simulink model "ModelRiki"  (R2020a)
settings: Solver=ode45  StartTime=0.0  StopTime=inf  MaxStep=Ts  RelTol=1e-3  EnableMultiTasking=on
model workspace (MAT data in the model file):
  CG : Simulink.Parameter (value not decoded)
  GPSLL : Simulink.Parameter (value not decoded)
  Inertia : Simulink.Parameter (value not decoded)
  Mass : Simulink.Parameter (value not decoded)
  Ts : Simulink.Parameter (value not decoded)
values from neighbouring files (symbols this model uses):
  AltKp = 0.03    [params.mat]
  AltRateBias = 0.65    [params.mat]
  AltRateKi = 0.01    [params.mat]
  AltRateKp = 0.05    [params.mat]
  AltRateMax = 6    [params.mat]
  FilterK = [0.01 0.01 0.01 0.01 0.01 0.01 0.01 0.01 0.01 0.01 0.01 0.01 ... (100 elements, 1x100)]    [params.mat]
  PosKp = 0.1    [params.mat]
  RollPitchKp = 10    [params.mat]
  RollPitchMax = 30    [params.mat]
  RollPitchRateKd = 5e-05    [params.mat]
  RollPitchRateKi = 0.002    [params.mat]
  RollPitchRateKp = 0.0007    [params.mat]
  RollPitchRateMax = 200    [params.mat]
  VelKi = 0.02    [params.mat]
  VelKp = 0.15    [params.mat]
  VelMax = 6    [params.mat]
  Waypts = [10 20 50 50 50 50 200 20 20 0 0 50 ... (27 elements, 9x3)]    [params.mat]
  YawKp = 3    [params.mat]
  YawRateKi = 0.000213867089849    [params.mat]
  YawRateKp = 0.00321759853461    [params.mat]
  YawRateMax = 180    [params.mat]
symbols that are objects in the model workspace (value not decoded): CG, Mass, Ts
undefined symbols (not defined in the file or in its folder): AltRateKd, DiscIntNeverNeededParam, Earth, Receive, Send, sigbuilder_block, WGS84
libraries: simulink x50, sharedutil x8, simulink_extras x7, aerolibfltsims x5, aerolibanimutils x2, aerolibtransform2 x2, aerolibconvert2 x2, shared6dof x1, aerolibatmos2 x1
(part 4 of 4)

== system ModelRiki/Model/Landing Gears/W2 Wheel ==
  Model BUS : Inport
  TerrainHeight : Inport  Port=2
  Add : Sum
  Add1 : Sum  Inputs=|++
  Bus Selector : BusSelector  OutputSignals=DCM,Xe
  Compare To Constant : simulink/Logic and Bit Operations/Compare To Constant  relop=>=  const=0  OutDataTypeStr=uint8
  Display : Display
  Display1 : Display
  Display2 : Display
  Enabled Subsystem : Subsystem  TreatAsAtomicUnit=on
  Gear Location (Body) : Constant  Value=WheelLoc
  Matrix Multiply : Product  Multiplication=Matrix(*)
  Reshape : Reshape  OutputDimensionality=Row vector (2-D)
  Selector : Selector  InputPortWidth=3  IndexOptions=Index vector (dialog)  Indices=[3]  OutputSizes=1
  M[Nm] : Outport
  F[N] : Outport  Port=2
  wires:
  TerrainHeight/1 -> Add1/2
  Add1/1 -> Compare To Constant/1, Enabled Subsystem/1(Height)
  Selector/1 -> Add1/1
  Model BUS/1 -> Bus Selector/1
  Enabled Subsystem/2(M[Nm]) -> Display2/1, M[Nm]/1
  Enabled Subsystem/1(F[N]) -> Display1/1, F[N]/1
  Compare To Constant/1 -> Enabled Subsystem/Enable
  Reshape/1 -> Matrix Multiply/1
  Add/1 -> Selector/1, Display/1  "locationNED"
  Matrix Multiply/1 -> Add/1
  Gear Location (Body)/1 -> Reshape/1
  Bus Selector/2 -> Add/2  "<Xe>"
  Bus Selector/1 -> Matrix Multiply/2  "<DCM>"

== system ModelRiki/Model/Landing Gears/W3 Wheel ==
  Model BUS : Inport
  TerrainHeight : Inport  Port=2
  Add : Sum
  Add1 : Sum  Inputs=|++
  Bus Selector : BusSelector  OutputSignals=DCM,Xe
  Compare To Constant : simulink/Logic and Bit Operations/Compare To Constant  relop=>=  const=0  OutDataTypeStr=uint8
  Display : Display
  Display1 : Display
  Display2 : Display
  Enabled Subsystem : Subsystem  TreatAsAtomicUnit=on
  Gear Location (Body) : Constant  Value=WheelLoc
  Matrix Multiply : Product  Multiplication=Matrix(*)
  Reshape : Reshape  OutputDimensionality=Row vector (2-D)
  Selector : Selector  InputPortWidth=3  IndexOptions=Index vector (dialog)  Indices=[3]  OutputSizes=1
  M[Nm] : Outport
  F[N] : Outport  Port=2
  wires:
  Bus Selector/1 -> Matrix Multiply/2  "<DCM>"
  Bus Selector/2 -> Add/2  "<Xe>"
  Gear Location (Body)/1 -> Reshape/1
  Matrix Multiply/1 -> Add/1
  Add/1 -> Display/1, Selector/1  "locationNED"
  Reshape/1 -> Matrix Multiply/1
  Compare To Constant/1 -> Enabled Subsystem/Enable
  Enabled Subsystem/1(F[N]) -> F[N]/1, Display1/1
  Enabled Subsystem/2(M[Nm]) -> M[Nm]/1, Display2/1
  Model BUS/1 -> Bus Selector/1
  Selector/1 -> Add1/1
  Add1/1 -> Enabled Subsystem/1(Height), Compare To Constant/1
  TerrainHeight/1 -> Add1/2

== system ModelRiki/Model/Landing Gears/W4 Wheel ==
  Model BUS : Inport
  TerrainHeight : Inport  Port=2
  Add : Sum
  Add1 : Sum  Inputs=|++
  Bus Selector : BusSelector  OutputSignals=DCM,Xe
  Compare To Constant : simulink/Logic and Bit Operations/Compare To Constant  relop=>=  const=0  OutDataTypeStr=uint8
  Display : Display
  Display1 : Display
  Display2 : Display
  Enabled Subsystem : Subsystem  TreatAsAtomicUnit=on
  Gear Location (Body) : Constant  Value=WheelLoc
  Matrix Multiply : Product  Multiplication=Matrix(*)
  Reshape : Reshape  OutputDimensionality=Row vector (2-D)
  Selector : Selector  InputPortWidth=3  IndexOptions=Index vector (dialog)  Indices=[3]  OutputSizes=1
  M[Nm] : Outport
  F[N] : Outport  Port=2
  wires:
  TerrainHeight/1 -> Add1/2
  Add1/1 -> Compare To Constant/1, Enabled Subsystem/1(Height)
  Selector/1 -> Add1/1
  Model BUS/1 -> Bus Selector/1
  Enabled Subsystem/2(M[Nm]) -> Display2/1, M[Nm]/1
  Enabled Subsystem/1(F[N]) -> Display1/1, F[N]/1
  Compare To Constant/1 -> Enabled Subsystem/Enable
  Reshape/1 -> Matrix Multiply/1
  Add/1 -> Selector/1, Display/1  "locationNED"
  Matrix Multiply/1 -> Add/1
  Gear Location (Body)/1 -> Reshape/1
  Bus Selector/2 -> Add/2  "<Xe>"
  Bus Selector/1 -> Matrix Multiply/2  "<DCM>"

== system ModelRiki/Model/Propulsion/Motor1 ==
  InputPWM : Inport
  3x3 Cross Product : sharedutil/3x3 Cross Product  aMode=aMode
      settings: SourceProductBaseCode=AE,PW,MT,VE,VP
  Add : Sum  Inputs=+-
  Add1 : Sum  Inputs=|++
  Constant1 : Constant  Value="[0.159 -0.159  -0.05]"
  Constant2 : Constant  Value=CG
  Product : Product  RndMeth=Zero
  Product1 : Product  RndMeth=Zero
  Subsystem : Subsystem
  Terminator1 : Terminator
  Vector : Constant  Value=[0 0 -1]
  Vector1 : Constant  Value=[0 0 -1.0]
  F[N] : Outport
  M[Nm] : Outport  Port=2
  Current[A] : Outport  Port=3
  wires:
  Vector/1 -> Product/1  "Forcevector"
  Product/1 -> 3x3 Cross Product/2, F[N]/1
  Add/1 -> 3x3 Cross Product/1  "r"
  Constant1/1 -> Add/1  "Position"
  Constant2/1 -> Add/2  "CG"
  Subsystem/1(Thrust) -> Product/2
  InputPWM/1 -> Subsystem/1(PWM)
  3x3 Cross Product/1 -> Add1/1  "M"
  Add1/1 -> M[Nm]/1
  Product1/1 -> Add1/2  "RotorTorque"
  Subsystem/2(Torque) -> Product1/2
  Vector1/1 -> Product1/1
  Subsystem/3(Current) -> Current[A]/1
  Subsystem/4(RPM) -> Terminator1/1

== system ModelRiki/Model/Propulsion/Motor2 ==
  InputPWM : Inport
  3x3 Cross Product : sharedutil/3x3 Cross Product  aMode=aMode
      settings: SourceProductBaseCode=AE,PW,MT,VE,VP
  Add : Sum  Inputs=+-
  Add1 : Sum  Inputs=|++
  Constant1 : Constant  Value="[0.159 0.159  -0.05]"
  Constant2 : Constant  Value=CG
  Product : Product  RndMeth=Zero
  Product1 : Product  RndMeth=Zero
  Subsystem : Subsystem
  Terminator1 : Terminator
  Vector : Constant  Value=[0 0 -1]
  Vector1 : Constant  Value=[0 0 1.0]
  F[N] : Outport
  M[Nm] : Outport  Port=2
  Current[A] : Outport  Port=3
  wires:
  Vector/1 -> Product/1  "Forcevector"
  Product/1 -> 3x3 Cross Product/2, F[N]/1
  Add/1 -> 3x3 Cross Product/1  "r"
  Constant1/1 -> Add/1  "Position"
  Constant2/1 -> Add/2  "CG"
  Subsystem/1(Thrust) -> Product/2
  InputPWM/1 -> Subsystem/1(PWM)
  3x3 Cross Product/1 -> Add1/1  "M"
  Add1/1 -> M[Nm]/1
  Product1/1 -> Add1/2  "RotorTorque"
  Subsystem/2(Torque) -> Product1/2
  Vector1/1 -> Product1/1
  Subsystem/3(Current) -> Current[A]/1
  Subsystem/4(RPM) -> Terminator1/1

== system ModelRiki/Model/Propulsion/Motor3 ==
  InputPWM : Inport
  3x3 Cross Product : sharedutil/3x3 Cross Product  aMode=aMode
      settings: SourceProductBaseCode=AE,PW,MT,VE,VP
  Add : Sum  Inputs=+-
  Add1 : Sum  Inputs=|++
  Constant1 : Constant  Value="[-0.159 0.159  -0.05]"
  Constant2 : Constant  Value=CG
  Product : Product  RndMeth=Zero
  Product1 : Product  RndMeth=Zero
  Subsystem : Subsystem
  Terminator1 : Terminator
  Vector : Constant  Value=[0 0 -1]
  Vector1 : Constant  Value=[0 0 -1.0]
  F[N] : Outport
  M[Nm] : Outport  Port=2
  Current[A] : Outport  Port=3
  wires:
  Vector/1 -> Product/1  "Forcevector"
  Product/1 -> 3x3 Cross Product/2, F[N]/1
  Add/1 -> 3x3 Cross Product/1  "r"
  Constant1/1 -> Add/1  "Position"
  Constant2/1 -> Add/2  "CG"
  Subsystem/1(Thrust) -> Product/2
  InputPWM/1 -> Subsystem/1(PWM)
  3x3 Cross Product/1 -> Add1/1  "M"
  Add1/1 -> M[Nm]/1
  Product1/1 -> Add1/2  "RotorTorque"
  Subsystem/2(Torque) -> Product1/2
  Vector1/1 -> Product1/1
  Subsystem/3(Current) -> Current[A]/1
  Subsystem/4(RPM) -> Terminator1/1

== system ModelRiki/Model/Propulsion/Motor4 ==
  InputPWM : Inport
  3x3 Cross Product : sharedutil/3x3 Cross Product  aMode=aMode
      settings: SourceProductBaseCode=AE,PW,MT,VE,VP
  Add : Sum  Inputs=+-
  Add1 : Sum  Inputs=|++
  Constant1 : Constant  Value="[-0.159 -0.159  -0.05]"
  Constant2 : Constant  Value=CG
  Product : Product  RndMeth=Zero
  Product1 : Product  RndMeth=Zero
  Subsystem : Subsystem
  Terminator1 : Terminator
  Vector : Constant  Value=[0 0 -1]
  Vector1 : Constant  Value=[0 0 1.0]
  F[N] : Outport
  M[Nm] : Outport  Port=2
  Current[A] : Outport  Port=3
  wires:
  Vector/1 -> Product/1  "Forcevector"
  Product/1 -> 3x3 Cross Product/2, F[N]/1
  Add/1 -> 3x3 Cross Product/1  "r"
  Constant1/1 -> Add/1  "Position"
  Constant2/1 -> Add/2  "CG"
  Subsystem/1(Thrust) -> Product/2
  InputPWM/1 -> Subsystem/1(PWM)
  3x3 Cross Product/1 -> Add1/1  "M"
  Add1/1 -> M[Nm]/1
  Product1/1 -> Add1/2  "RotorTorque"
  Subsystem/2(Torque) -> Product1/2
  Vector1/1 -> Product1/1
  Subsystem/3(Current) -> Current[A]/1
  Subsystem/4(RPM) -> Terminator1/1

== system ModelRiki/Ctrl/AutoCtrl/Mapper/LimitAndRescale ==
  Scaled : Inport
  Constant : Constant  Value=1100  OutDataTypeStr=single
  Gain : Gain  Gain=(1900-1100)
  Limit3 : Saturate  UpperLimit=1  LowerLimit=0
  Subtract : Sum
  ESCPWM : Outport
  wires:
  Constant/1 -> Subtract/2
  Gain/1 -> Subtract/1
  Scaled/1 -> Limit3/1
  Subtract/1 -> ESCPWM/1
  Limit3/1 -> Gain/1

== system ModelRiki/Ctrl/AutoCtrl/Mapper/LimitAndRescale1 ==
  Scaled : Inport
  Constant : Constant  Value=1100  OutDataTypeStr=single
  Gain : Gain  Gain=(1900-1100)
  Limit3 : Saturate  UpperLimit=1  LowerLimit=0
  Subtract : Sum
  ESCPWM : Outport
  wires:
  Constant/1 -> Subtract/2
  Gain/1 -> Subtract/1
  Scaled/1 -> Limit3/1
  Subtract/1 -> ESCPWM/1
  Limit3/1 -> Gain/1

== system ModelRiki/Ctrl/AutoCtrl/Mapper/LimitAndRescale2 ==
  Scaled : Inport
  Constant : Constant  Value=1100  OutDataTypeStr=single
  Gain : Gain  Gain=(1900-1100)
  Limit3 : Saturate  UpperLimit=1  LowerLimit=0
  Subtract : Sum
  ESCPWM : Outport
  wires:
  Constant/1 -> Subtract/2
  Gain/1 -> Subtract/1
  Scaled/1 -> Limit3/1
  Subtract/1 -> ESCPWM/1
  Limit3/1 -> Gain/1

== system ModelRiki/Ctrl/AutoCtrl/Mapper/LimitAndRescale3 ==
  Scaled : Inport
  Constant : Constant  Value=1100  OutDataTypeStr=single
  Gain : Gain  Gain=(1900-1100)
  Limit3 : Saturate  UpperLimit=1  LowerLimit=0
  Subtract : Sum
  ESCPWM : Outport
  wires:
  Constant/1 -> Subtract/2
  Gain/1 -> Subtract/1
  Scaled/1 -> Limit3/1
  Subtract/1 -> ESCPWM/1
  Limit3/1 -> Gain/1

== system ModelRiki/Ctrl/ManualCtrl/Mapper/LimitAndRescale ==
  Scaled : Inport
  Constant : Constant  Value=1100  OutDataTypeStr=single
  Gain : Gain  Gain=(1900-1100)
  Limit3 : Saturate  UpperLimit=1  LowerLimit=0
  Subtract : Sum
  ESCPWM : Outport
  wires:
  Constant/1 -> Subtract/2
  Gain/1 -> Subtract/1
  Scaled/1 -> Limit3/1
  Subtract/1 -> ESCPWM/1
  Limit3/1 -> Gain/1

== system ModelRiki/Ctrl/ManualCtrl/Mapper/LimitAndRescale1 ==
  Scaled : Inport
  Constant : Constant  Value=1100  OutDataTypeStr=single
  Gain : Gain  Gain=(1900-1100)
  Limit3 : Saturate  UpperLimit=1  LowerLimit=0
  Subtract : Sum
  ESCPWM : Outport
  wires:
  Constant/1 -> Subtract/2
  Gain/1 -> Subtract/1
  Scaled/1 -> Limit3/1
  Subtract/1 -> ESCPWM/1
  Limit3/1 -> Gain/1

== system ModelRiki/Ctrl/ManualCtrl/Mapper/LimitAndRescale2 ==
  Scaled : Inport
  Constant : Constant  Value=1100  OutDataTypeStr=single
  Gain : Gain  Gain=(1900-1100)
  Limit3 : Saturate  UpperLimit=1  LowerLimit=0
  Subtract : Sum
  ESCPWM : Outport
  wires:
  Constant/1 -> Subtract/2
  Gain/1 -> Subtract/1
  Scaled/1 -> Limit3/1
  Subtract/1 -> ESCPWM/1
  Limit3/1 -> Gain/1

== system ModelRiki/Ctrl/ManualCtrl/Mapper/LimitAndRescale3 ==
  Scaled : Inport
  Constant : Constant  Value=1100  OutDataTypeStr=single
  Gain : Gain  Gain=(1900-1100)
  Limit3 : Saturate  UpperLimit=1  LowerLimit=0
  Subtract : Sum
  ESCPWM : Outport
  wires:
  Constant/1 -> Subtract/2
  Gain/1 -> Subtract/1
  Scaled/1 -> Limit3/1
  Subtract/1 -> ESCPWM/1
  Limit3/1 -> Gain/1

== system ModelRiki/Ctrl/RateCtrl/Mapper/LimitAndRescale ==
  Scaled : Inport
  Constant : Constant  Value=1100  OutDataTypeStr=single
  Gain : Gain  Gain=(1900-1100)
  Limit3 : Saturate  UpperLimit=1  LowerLimit=0
  Subtract : Sum
  ESCPWM : Outport
  wires:
  Constant/1 -> Subtract/2
  Gain/1 -> Subtract/1
  Scaled/1 -> Limit3/1
  Subtract/1 -> ESCPWM/1
  Limit3/1 -> Gain/1

== system ModelRiki/Ctrl/RateCtrl/Mapper/LimitAndRescale1 ==
  Scaled : Inport
  Constant : Constant  Value=1100  OutDataTypeStr=single
  Gain : Gain  Gain=(1900-1100)
  Limit3 : Saturate  UpperLimit=1  LowerLimit=0
  Subtract : Sum
  ESCPWM : Outport
  wires:
  Constant/1 -> Subtract/2
  Gain/1 -> Subtract/1
  Scaled/1 -> Limit3/1
  Subtract/1 -> ESCPWM/1
  Limit3/1 -> Gain/1

== system ModelRiki/Ctrl/RateCtrl/Mapper/LimitAndRescale2 ==
  Scaled : Inport
  Constant : Constant  Value=1100  OutDataTypeStr=single
  Gain : Gain  Gain=(1900-1100)
  Limit3 : Saturate  UpperLimit=1  LowerLimit=0
  Subtract : Sum
  ESCPWM : Outport
  wires:
  Constant/1 -> Subtract/2
  Gain/1 -> Subtract/1
  Scaled/1 -> Limit3/1
  Subtract/1 -> ESCPWM/1
  Limit3/1 -> Gain/1

== system ModelRiki/Ctrl/RateCtrl/Mapper/LimitAndRescale3 ==
  Scaled : Inport
  Constant : Constant  Value=1100  OutDataTypeStr=single
  Gain : Gain  Gain=(1900-1100)
  Limit3 : Saturate  UpperLimit=1  LowerLimit=0
  Subtract : Sum
  ESCPWM : Outport
  wires:
  Constant/1 -> Subtract/2
  Gain/1 -> Subtract/1
  Scaled/1 -> Limit3/1
  Subtract/1 -> ESCPWM/1
  Limit3/1 -> Gain/1

== system ModelRiki/Ctrl/RollPitchCtrl/Mapper/LimitAndRescale ==
  Scaled : Inport
  Constant : Constant  Value=1100  OutDataTypeStr=single
  Gain : Gain  Gain=(1900-1100)
  Limit3 : Saturate  UpperLimit=1  LowerLimit=0
  Subtract : Sum
  ESCPWM : Outport
  wires:
  Constant/1 -> Subtract/2
  Gain/1 -> Subtract/1
  Scaled/1 -> Limit3/1
  Subtract/1 -> ESCPWM/1
  Limit3/1 -> Gain/1

== system ModelRiki/Ctrl/RollPitchCtrl/Mapper/LimitAndRescale1 ==
  Scaled : Inport
  Constant : Constant  Value=1100  OutDataTypeStr=single
  Gain : Gain  Gain=(1900-1100)
  Limit3 : Saturate  UpperLimit=1  LowerLimit=0
  Subtract : Sum
  ESCPWM : Outport
  wires:
  Constant/1 -> Subtract/2
  Gain/1 -> Subtract/1
  Scaled/1 -> Limit3/1
  Subtract/1 -> ESCPWM/1
  Limit3/1 -> Gain/1

== system ModelRiki/Ctrl/RollPitchCtrl/Mapper/LimitAndRescale2 ==
  Scaled : Inport
  Constant : Constant  Value=1100  OutDataTypeStr=single
  Gain : Gain  Gain=(1900-1100)
  Limit3 : Saturate  UpperLimit=1  LowerLimit=0
  Subtract : Sum
  ESCPWM : Outport
  wires:
  Constant/1 -> Subtract/2
  Gain/1 -> Subtract/1
  Scaled/1 -> Limit3/1
  Subtract/1 -> ESCPWM/1
  Limit3/1 -> Gain/1

== system ModelRiki/Ctrl/RollPitchCtrl/Mapper/LimitAndRescale3 ==
  Scaled : Inport
  Constant : Constant  Value=1100  OutDataTypeStr=single
  Gain : Gain  Gain=(1900-1100)
  Limit3 : Saturate  UpperLimit=1  LowerLimit=0
  Subtract : Sum
  ESCPWM : Outport
  wires:
  Constant/1 -> Subtract/2
  Gain/1 -> Subtract/1
  Scaled/1 -> Limit3/1
  Subtract/1 -> ESCPWM/1
  Limit3/1 -> Gain/1

== system ModelRiki/Ctrl/VelocityCtrl/Mapper/LimitAndRescale ==
  Scaled : Inport
  Constant : Constant  Value=1100  OutDataTypeStr=single
  Gain : Gain  Gain=(1900-1100)
  Limit3 : Saturate  UpperLimit=1  LowerLimit=0
  Subtract : Sum
  ESCPWM : Outport
  wires:
  Constant/1 -> Subtract/2
  Gain/1 -> Subtract/1
  Scaled/1 -> Limit3/1
  Subtract/1 -> ESCPWM/1
  Limit3/1 -> Gain/1

== system ModelRiki/Ctrl/VelocityCtrl/Mapper/LimitAndRescale1 ==
  Scaled : Inport
  Constant : Constant  Value=1100  OutDataTypeStr=single
  Gain : Gain  Gain=(1900-1100)
  Limit3 : Saturate  UpperLimit=1  LowerLimit=0
  Subtract : Sum
  ESCPWM : Outport
  wires:
  Constant/1 -> Subtract/2
  Gain/1 -> Subtract/1
  Scaled/1 -> Limit3/1
  Subtract/1 -> ESCPWM/1
  Limit3/1 -> Gain/1

== system ModelRiki/Ctrl/VelocityCtrl/Mapper/LimitAndRescale2 ==
  Scaled : Inport
  Constant : Constant  Value=1100  OutDataTypeStr=single
  Gain : Gain  Gain=(1900-1100)
  Limit3 : Saturate  UpperLimit=1  LowerLimit=0
  Subtract : Sum
  ESCPWM : Outport
  wires:
  Constant/1 -> Subtract/2
  Gain/1 -> Subtract/1
  Scaled/1 -> Limit3/1
  Subtract/1 -> ESCPWM/1
  Limit3/1 -> Gain/1

== system ModelRiki/Ctrl/VelocityCtrl/Mapper/LimitAndRescale3 ==
  Scaled : Inport
  Constant : Constant  Value=1100  OutDataTypeStr=single
  Gain : Gain  Gain=(1900-1100)
  Limit3 : Saturate  UpperLimit=1  LowerLimit=0
  Subtract : Sum
  ESCPWM : Outport
  wires:
  Constant/1 -> Subtract/2
  Gain/1 -> Subtract/1
  Scaled/1 -> Limit3/1
  Subtract/1 -> ESCPWM/1
  Limit3/1 -> Gain/1

== system ModelRiki/Model/Landing Gears/W1 Wheel/Enabled Subsystem ==
  Height : Inport
  Enable : EnablePort
  3x3 Cross Product : sharedutil/3x3 Cross Product  aMode=aMode
      settings: SourceProductBaseCode=AE,PW,MT,VE,VP
  Add : Sum  Inputs=+-
  Add1 : Sum
  Constant2 : Constant  Value=CG
  Derivative : Derivative
  Gain : Gain  Gain=1000
  Gain1 : Gain  Gain=200
  Gear Location (Body) : Constant  Value=WheelLoc
  Gear Vector (up) : Constant  Value=[0 0 -1]
  Product : Product  RndMeth=Zero
  F[N] : Outport  OutputWhenDisabled=reset  InitialOutput=[0 0 0]
  M[Nm] : Outport  Port=2  OutputWhenDisabled=reset  InitialOutput=[0 0 0]
  wires:
  Product/1 -> 3x3 Cross Product/2, F[N]/1
  Add/1 -> 3x3 Cross Product/1  "r"
  Gear Location (Body)/1 -> Add/1  "Position"
  Constant2/1 -> Add/2  "CG"
  Gear Vector (up)/1 -> Product/1
  3x3 Cross Product/1 -> M[Nm]/1  "M"
  Height/1 -> Gain/1, Derivative/1
  Add1/1 -> Product/2
  Gain/1 -> Add1/1
  Derivative/1 -> Gain1/1
  Gain1/1 -> Add1/2

== system ModelRiki/Model/Landing Gears/W2 Wheel/Enabled Subsystem ==
  Height : Inport
  Enable : EnablePort
  3x3 Cross Product : sharedutil/3x3 Cross Product  aMode=aMode
      settings: SourceProductBaseCode=AE,PW,MT,VE,VP
  Add : Sum  Inputs=+-
  Add1 : Sum
  Constant2 : Constant  Value=CG
  Derivative : Derivative
  Gain : Gain  Gain=1000
  Gain1 : Gain  Gain=200
  Gear Location (Body) : Constant  Value=WheelLoc
  Gear Vector (up) : Constant  Value=[0 0 -1]
  Product : Product  RndMeth=Zero
  F[N] : Outport  OutputWhenDisabled=reset  InitialOutput=[0 0 0]
  M[Nm] : Outport  Port=2  OutputWhenDisabled=reset  InitialOutput=[0 0 0]
  wires:
  Gain1/1 -> Add1/2
  Derivative/1 -> Gain1/1
  Gain/1 -> Add1/1
  Add1/1 -> Product/2
  Height/1 -> Derivative/1, Gain/1
  3x3 Cross Product/1 -> M[Nm]/1  "M"
  Gear Vector (up)/1 -> Product/1
  Constant2/1 -> Add/2  "CG"
  Gear Location (Body)/1 -> Add/1  "Position"
  Add/1 -> 3x3 Cross Product/1  "r"
  Product/1 -> F[N]/1, 3x3 Cross Product/2

== system ModelRiki/Model/Landing Gears/W3 Wheel/Enabled Subsystem ==
  Height : Inport
  Enable : EnablePort
  3x3 Cross Product : sharedutil/3x3 Cross Product  aMode=aMode
      settings: SourceProductBaseCode=AE,PW,MT,VE,VP
  Add : Sum  Inputs=+-
  Add1 : Sum
  Constant2 : Constant  Value=CG
  Derivative : Derivative
  Gain : Gain  Gain=1000
  Gain1 : Gain  Gain=200
  Gear Location (Body) : Constant  Value=WheelLoc
  Gear Vector (up) : Constant  Value=[0 0 -1]
  Product : Product  RndMeth=Zero
  F[N] : Outport  OutputWhenDisabled=reset  InitialOutput=[0 0 0]
  M[Nm] : Outport  Port=2  OutputWhenDisabled=reset  InitialOutput=[0 0 0]
  wires:
  Product/1 -> 3x3 Cross Product/2, F[N]/1
  Add/1 -> 3x3 Cross Product/1  "r"
  Gear Location (Body)/1 -> Add/1  "Position"
  Constant2/1 -> Add/2  "CG"
  Gear Vector (up)/1 -> Product/1
  3x3 Cross Product/1 -> M[Nm]/1  "M"
  Height/1 -> Gain/1, Derivative/1
  Add1/1 -> Product/2
  Gain/1 -> Add1/1
  Derivative/1 -> Gain1/1
  Gain1/1 -> Add1/2

== system ModelRiki/Model/Landing Gears/W4 Wheel/Enabled Subsystem ==
  Height : Inport
  Enable : EnablePort
  3x3 Cross Product : sharedutil/3x3 Cross Product  aMode=aMode
      settings: SourceProductBaseCode=AE,PW,MT,VE,VP
  Add : Sum  Inputs=+-
  Add1 : Sum
  Constant2 : Constant  Value=CG
  Derivative : Derivative
  Gain : Gain  Gain=1000
  Gain1 : Gain  Gain=200
  Gear Location (Body) : Constant  Value=WheelLoc
  Gear Vector (up) : Constant  Value=[0 0 -1]
  Product : Product  RndMeth=Zero
  F[N] : Outport  OutputWhenDisabled=reset  InitialOutput=[0 0 0]
  M[Nm] : Outport  Port=2  OutputWhenDisabled=reset  InitialOutput=[0 0 0]
  wires:
  Gain1/1 -> Add1/2
  Derivative/1 -> Gain1/1
  Gain/1 -> Add1/1
  Add1/1 -> Product/2
  Height/1 -> Derivative/1, Gain/1
  3x3 Cross Product/1 -> M[Nm]/1  "M"
  Gear Vector (up)/1 -> Product/1
  Constant2/1 -> Add/2  "CG"
  Gear Location (Body)/1 -> Add/1  "Position"
  Add/1 -> 3x3 Cross Product/1  "r"
  Product/1 -> F[N]/1, 3x3 Cross Product/2

== system ModelRiki/Model/Propulsion/Motor1/Subsystem ==
  note: [N]
  note: [g]
  note: [Nm]
  note: [A]
  note: [20ms delay?]
  note: [Torque estimated]
  note: [1000-1900]
  note: Current
  note: Enable [>1150]
  PWM : Inport  OutDataTypeStr=double  PortDimensions=1  SampleTime=0
  Compare To Constant1 : simulink/Logic and Bit Operations/Compare To Constant  relop=>=  const=1150  OutDataTypeStr=boolean
  Constant1 : Constant  Value=0
  Gain2 : Gain  Gain=1/1000
  Gain3 : Gain  Gain=1/1000*9.81
  Polynomial4 : Polyval  Coefs="[194.0242  232.6928 -846.8342  374.2523]"
  Polynomial5 : Polyval  Coefs="[23.1858  -80.9421   97.9875  -40.9978]"
  Polynomial6 : Polyval  Coefs="1.0e+04 *[-0.6016    2.6561   -2.8627    0.8887]"
  Polynomial7 : Polyval  Coefs="1e-3*0.11*[194.0242  232.6928 -846.8342  374.2523]"
  Saturation1 : Saturate  UpperLimit=1900  LowerLimit=1000
  Switch{4..7} (4 alike) : Switch  Criteria=u2 ~= 0
  Transfer Fcn1 : TransferFcn  Denominator=[0.045 1]
  Transport Delay1 : TransportDelay  DelayTime=0.02
  Thrust : Outport  OutDataTypeStr=double  PortDimensions=1  SampleTime=0
  Torque : Outport  Port=2  OutDataTypeStr=double  PortDimensions=1  SampleTime=0
  Current : Outport  Port=3  OutDataTypeStr=double  PortDimensions=1  SampleTime=0
  RPM : Outport  Port=4  OutDataTypeStr=double  PortDimensions=1  SampleTime=0
  wires:
  Gain3/1 -> Thrust/1  "Thrust"
  Saturation1/1 -> Transport Delay1/1
  Transport Delay1/1 -> Transfer Fcn1/1
  Gain2/1 -> Polynomial4/1, Polynomial6/1, Polynomial5/1, Polynomial7/1
  Compare To Constant1/1 -> Switch4/2, Switch6/2, Switch5/2, Switch7/2
  Polynomial4/1 -> Switch4/1
  Constant1/1 -> Switch4/3, Switch6/3, Switch5/3, Switch7/3
  Switch4/1 -> Gain3/1  "Thrust"
  Polynomial5/1 -> Switch5/1
  Switch5/1 -> Current/1
  Polynomial6/1 -> Switch6/1
  Switch6/1 -> RPM/1  "RPM"
  Polynomial7/1 -> Switch7/1
  Switch7/1 -> Torque/1  "Torque"
  Transfer Fcn1/1 -> Gain2/1, Compare To Constant1/1
  PWM/1 -> Saturation1/1

== system ModelRiki/Model/Propulsion/Motor2/Subsystem ==
  note: [N]
  note: [g]
  note: [Nm]
  note: [A]
  note: [20ms delay?]
  note: [Torque estimated]
  note: [1000-1900]
  note: Current
  note: Enable [>1150]
  PWM : Inport  OutDataTypeStr=double  PortDimensions=1  SampleTime=0
  Compare To Constant1 : simulink/Logic and Bit Operations/Compare To Constant  relop=>=  const=1150  OutDataTypeStr=boolean
  Constant1 : Constant  Value=0
  Gain2 : Gain  Gain=1/1000
  Gain3 : Gain  Gain=1/1000*9.81
  Polynomial4 : Polyval  Coefs="[194.0242  232.6928 -846.8342  374.2523]"
  Polynomial5 : Polyval  Coefs="[23.1858  -80.9421   97.9875  -40.9978]"
  Polynomial6 : Polyval  Coefs="1.0e+04 *[-0.6016    2.6561   -2.8627    0.8887]"
  Polynomial7 : Polyval  Coefs="1e-3*0.11*[194.0242  232.6928 -846.8342  374.2523]"
  Saturation1 : Saturate  UpperLimit=1900  LowerLimit=1000
  Switch{4..7} (4 alike) : Switch  Criteria=u2 ~= 0
  Transfer Fcn1 : TransferFcn  Denominator=[0.045 1]
  Transport Delay1 : TransportDelay  DelayTime=0.02
  Thrust : Outport  OutDataTypeStr=double  PortDimensions=1  SampleTime=0
  Torque : Outport  Port=2  OutDataTypeStr=double  PortDimensions=1  SampleTime=0
  Current : Outport  Port=3  OutDataTypeStr=double  PortDimensions=1  SampleTime=0
  RPM : Outport  Port=4  OutDataTypeStr=double  PortDimensions=1  SampleTime=0
  wires:
  Gain3/1 -> Thrust/1  "Thrust"
  Saturation1/1 -> Transport Delay1/1
  Transport Delay1/1 -> Transfer Fcn1/1
  Gain2/1 -> Polynomial4/1, Polynomial6/1, Polynomial5/1, Polynomial7/1
  Compare To Constant1/1 -> Switch4/2, Switch6/2, Switch5/2, Switch7/2
  Polynomial4/1 -> Switch4/1
  Constant1/1 -> Switch4/3, Switch6/3, Switch5/3, Switch7/3
  Switch4/1 -> Gain3/1  "Thrust"
  Polynomial5/1 -> Switch5/1
  Switch5/1 -> Current/1
  Polynomial6/1 -> Switch6/1
  Switch6/1 -> RPM/1  "RPM"
  Polynomial7/1 -> Switch7/1
  Switch7/1 -> Torque/1  "Torque"
  Transfer Fcn1/1 -> Gain2/1, Compare To Constant1/1
  PWM/1 -> Saturation1/1

== system ModelRiki/Model/Propulsion/Motor3/Subsystem ==
  note: [N]
  note: [g]
  note: [Nm]
  note: [A]
  note: [20ms delay?]
  note: [Torque estimated]
  note: [1000-1900]
  note: Current
  note: Enable [>1150]
  PWM : Inport  OutDataTypeStr=double  PortDimensions=1  SampleTime=0
  Compare To Constant1 : simulink/Logic and Bit Operations/Compare To Constant  relop=>=  const=1150  OutDataTypeStr=boolean
  Constant1 : Constant  Value=0
  Gain2 : Gain  Gain=1/1000
  Gain3 : Gain  Gain=1/1000*9.81
  Polynomial4 : Polyval  Coefs="[194.0242  232.6928 -846.8342  374.2523]"
  Polynomial5 : Polyval  Coefs="[23.1858  -80.9421   97.9875  -40.9978]"
  Polynomial6 : Polyval  Coefs="1.0e+04 *[-0.6016    2.6561   -2.8627    0.8887]"
  Polynomial7 : Polyval  Coefs="1e-3*0.11*[194.0242  232.6928 -846.8342  374.2523]"
  Saturation1 : Saturate  UpperLimit=1900  LowerLimit=1000
  Switch{4..7} (4 alike) : Switch  Criteria=u2 ~= 0
  Transfer Fcn1 : TransferFcn  Denominator=[0.045 1]
  Transport Delay1 : TransportDelay  DelayTime=0.02
  Thrust : Outport  OutDataTypeStr=double  PortDimensions=1  SampleTime=0
  Torque : Outport  Port=2  OutDataTypeStr=double  PortDimensions=1  SampleTime=0
  Current : Outport  Port=3  OutDataTypeStr=double  PortDimensions=1  SampleTime=0
  RPM : Outport  Port=4  OutDataTypeStr=double  PortDimensions=1  SampleTime=0
  wires:
  Gain3/1 -> Thrust/1  "Thrust"
  Saturation1/1 -> Transport Delay1/1
  Transport Delay1/1 -> Transfer Fcn1/1
  Gain2/1 -> Polynomial4/1, Polynomial6/1, Polynomial5/1, Polynomial7/1
  Compare To Constant1/1 -> Switch4/2, Switch6/2, Switch5/2, Switch7/2
  Polynomial4/1 -> Switch4/1
  Constant1/1 -> Switch4/3, Switch6/3, Switch5/3, Switch7/3
  Switch4/1 -> Gain3/1  "Thrust"
  Polynomial5/1 -> Switch5/1
  Switch5/1 -> Current/1
  Polynomial6/1 -> Switch6/1
  Switch6/1 -> RPM/1  "RPM"
  Polynomial7/1 -> Switch7/1
  Switch7/1 -> Torque/1  "Torque"
  Transfer Fcn1/1 -> Gain2/1, Compare To Constant1/1
  PWM/1 -> Saturation1/1

== system ModelRiki/Model/Propulsion/Motor4/Subsystem ==
  note: [N]
  note: [g]
  note: [Nm]
  note: [A]
  note: [20ms delay?]
  note: [Torque estimated]
  note: [1000-1900]
  note: Current
  note: Enable [>1150]
  PWM : Inport  OutDataTypeStr=double  PortDimensions=1  SampleTime=0
  Compare To Constant1 : simulink/Logic and Bit Operations/Compare To Constant  relop=>=  const=1150  OutDataTypeStr=boolean
  Constant1 : Constant  Value=0
  Gain2 : Gain  Gain=1/1000
  Gain3 : Gain  Gain=1/1000*9.81
  Polynomial4 : Polyval  Coefs="[194.0242  232.6928 -846.8342  374.2523]"
  Polynomial5 : Polyval  Coefs="[23.1858  -80.9421   97.9875  -40.9978]"
  Polynomial6 : Polyval  Coefs="1.0e+04 *[-0.6016    2.6561   -2.8627    0.8887]"
  Polynomial7 : Polyval  Coefs="1e-3*0.11*[194.0242  232.6928 -846.8342  374.2523]"
  Saturation1 : Saturate  UpperLimit=1900  LowerLimit=1000
  Switch{4..7} (4 alike) : Switch  Criteria=u2 ~= 0
  Transfer Fcn1 : TransferFcn  Denominator=[0.045 1]
  Transport Delay1 : TransportDelay  DelayTime=0.02
  Thrust : Outport  OutDataTypeStr=double  PortDimensions=1  SampleTime=0
  Torque : Outport  Port=2  OutDataTypeStr=double  PortDimensions=1  SampleTime=0
  Current : Outport  Port=3  OutDataTypeStr=double  PortDimensions=1  SampleTime=0
  RPM : Outport  Port=4  OutDataTypeStr=double  PortDimensions=1  SampleTime=0
  wires:
  Gain3/1 -> Thrust/1  "Thrust"
  Saturation1/1 -> Transport Delay1/1
  Transport Delay1/1 -> Transfer Fcn1/1
  Gain2/1 -> Polynomial4/1, Polynomial6/1, Polynomial5/1, Polynomial7/1
  Compare To Constant1/1 -> Switch4/2, Switch6/2, Switch5/2, Switch7/2
  Polynomial4/1 -> Switch4/1
  Constant1/1 -> Switch4/3, Switch6/3, Switch5/3, Switch7/3
  Switch4/1 -> Gain3/1  "Thrust"
  Polynomial5/1 -> Switch5/1
  Switch5/1 -> Current/1
  Polynomial6/1 -> Switch6/1
  Switch6/1 -> RPM/1  "RPM"
  Polynomial7/1 -> Switch7/1
  Switch7/1 -> Torque/1  "Torque"
  Transfer Fcn1/1 -> Gain2/1, Compare To Constant1/1
  PWM/1 -> Saturation1/1

== stateflow chart ModelRiki/Ctrl/Chart ==
  settings: updateMethod=DISCRETE  sampleTime=Ts
  state SystemLogic [parallel]
    en: Mode = uint8(0);
    du: SelectMode()
    settings: executionOrder=1
    state On
      en:
      ModeOld = Mode;
      state ManualMode
        entry:
        ActualMode=uint8(1);
      state RateMode
        entry:
        ActualMode=uint8(2);
      state RollPitchMode
        entry:
        ActualMode=uint8(3);
      state VelocityMode
        entry:
        ActualMode=uint8(4);
      state AutoMode
        state InitSegment
          entry:
          ActualMode=10+wayIndex;
          CalculateTrajSegment(wayIndex,wayIndex+1, TrajZNEVParams(4))
          Time = single(0);
          AutoRefAng = atan2(Waypoints(wayIndex+1,3)-Waypoints(wayIndex,3), Waypoints(wayIndex+1,2)-Waypoints(wayIndex,2) );
        state Idle
          entry:
          wayIndex = uint8(1);
          ActualMode=uint8(5);
          during:
          AutoRef=Waypoints(1,:); % Altitude, N, E
          AutoRefAng = single(-2000); % disable
        state GotoWaypoint
          during:
          AutoRef = P1 + dPdT*Time;
          Time = Time+Ts;
        state NextWaypoint
          entry:
          wayIndex=wayIndex+1;
        state End
        state Orbit
          during:
          AutoRef(1) = TrajZNEVParams(1);
          AutoRef(2) = TrajZNEVParams(2) + cos(OrbPhi) * OrbRadius;
          AutoRef(3) = TrajZNEVParams(3) + sin(OrbPhi) * OrbRadius;
          OrbPhi = OrbPhi+(OrbdPhidT*Ts);
          AutoRefAng = OrbPhi+pi;
          while AutoRefAng > 2*pi
          AutoRefAng = AutoRefAng-(2*pi);
          end
        state InitOrbitBezSecera
          entry:
          OrbRadius = sqrt( (Position(2) - TrajZNEVParams(2))^2 + (Position(3) - TrajZNEVParams(3))^2 );
          OrbPhi = atan2((Position(3) - TrajZNEVParams(3)), (Position(2) - TrajZNEVParams(2)));
          OrbdPhidT = TrajZNEVParams(4) / OrbRadius; % phi per second to match speed V
        GotoWaypoint -> Idle [order 2] : [ExecuteWaypoints == 10] % Abort Command
        (default) -> Idle
        InitSegment -> GotoWaypoint
        Idle -> InitSegment [order 1] : [ ExecuteWaypoints == 1 && (WayCnt > 0) ]
        Idle -> InitOrbitBezSecera [order 2] : [ ExecuteWaypoints == 2]
        GotoWaypoint -> NextWaypoint [order 1] : [Time > Ttotal]
        End -> Idle
        (junction 284) -> InitSegment [order 2]
        (junction 284) -> End [order 1] : [wayIndex > WayCnt]
        NextWaypoint -> (junction 284) : [ after(1000, tick)]
            | % Optional delay
        InitOrbitBezSecera -> Orbit
    state Off
      entry:
      ActualMode=uint8(0);
    state SelectMode [function]
      (default) -> (junction 319)
      (junction 319) -> (junction 314) [order 1] : [ActualMode > 10]
      (junction 319) -> (junction 188) [order 2]
      (junction 314) -> (junction 182)
      (junction 188) -> (junction 179) [order 1] : [Throttle < 400 && Mode~=5]
      (junction 179) -> (junction 182) : {Mode = uint8(0);}
      (junction 188) -> (junction 218) [order 2]
      (junction 182) -> (junction 226)
      (junction 218) -> (junction 215) [order 1] : [ ModeInput < 600 ]
      (junction 215) -> (junction 226) : {Mode = ModeCode;}
      (junction 218) -> (junction 220) [order 2]
      (junction 226) -> (junction 228)
      (junction 220) -> (junction 221) [order 1] : [ ModeInput < 1300 ]
      (junction 221) -> (junction 228) : {Mode = uint8(4);}
      (junction 220) -> (junction 216) [order 2] : {Mode = uint8(5);}
      (junction 228) -> (junction 233)
      (junction 233) -> (junction 216)
      (junction 216) -> (junction 180)
    (default) -> SystemLogic.Off
    SystemLogic.Off -> ManualMode [order 1] : [Mode==1]
    SystemLogic.Off -> RateMode [order 2] : [Mode==2]
    SystemLogic.Off -> RollPitchMode [order 3] : [Mode==3]
    SystemLogic.Off -> VelocityMode [order 4] : [Mode==4]
    SystemLogic.Off -> AutoMode [order 5] : [Mode==5]
    SystemLogic.On -> SystemLogic.Off : [ Mode ~= ModeOld ]
  state LEDs [parallel]
    settings: executionOrder=2
    state Off
      en:
      LEDs(1) = false;
      LEDs(2) = false;
      LEDs(3) = false;
      state RedOn
        entry: LEDs(1) = true;
      state RedOff
        entry: LEDs(1) = false;
      (default) -> RedOn
      RedOn -> RedOff : [after(100,tick)]
      RedOff -> RedOn : [after(100,tick)]
    state On
      en:
      LEDs(1) = false;
      LEDs(2) = false;
      LEDs(3) = false;
      state GreenOn
        entry: LEDs(2) = true;
      state GreenOff
        entry: LEDs(2) = false;
      (default) -> GreenOn
      GreenOn -> GreenOff : [after(100,tick)]
      GreenOff -> GreenOn : [after(100,tick)]
    (default) -> LEDs.Off
    LEDs.Off -> LEDs.On : [in(SystemLogic.On)]
    LEDs.On -> LEDs.Off : [in(SystemLogic.Off)]
  data: index1 function_input uint8 size=1; index2 function_input uint8 size=1; velocity function_input single size=1; OrbPhi local single size=1; OrbRadius local single size=1; OrbdPhidT local single size=1; dPdT local single size=[1 3]; P1 local single size=[1 3]; Ttotal local single size=1; Time local single size=1; ActualMode output uint8; LEDs output boolean size=3; Mode local uint8; Throttle input single; Off output boolean; ManualMode output boolean; RateMode output boolean; RollPitchMode output boolean; ModeInput input uint32; VelocityMode output boolean; AutoMode output boolean; ModeCode input uint8; Waypoints input single size=[9 3]; wayIndex local uint8; Position input single size=[3]; WayCnt input int32; ExecuteWaypoints input uint32; TrajZNEVParams input single size=4; Ts constant single =Ts; AutoRef output single size=[1 3]; AutoRefAng output single size=1; ModeOld local uint8 size=1
  function CalculateTrajSegment(index1, index2, velocity ):
    | function CalculateTrajSegment(index1, index2, velocity )
    | P1=Waypoints(index1,:);
    | P2=Waypoints(index2,:);
    | dP=P2-P1;
    | dPLen = norm(dP);
    | Ttotal = dPLen/velocity;
    | dPdT=dP/Ttotal;

== matlab function ModelRiki/Ctrl/VelocityCtrl/Yaw Controller/Correct Yaw1 ==
  data: u input; y output
function y = fcn(u)
%#codegen
y = mod(u, 360);
if y > 180  
    y=y-360;
end

== matlab function ModelRiki/Ctrl/AutoCtrl/Yaw Controller/Correct Yaw1 ==
  data: u input; y output
function y = fcn(u)
%#codegen
y = mod(u, 360);
if y > 180  
    y=y-360;
end

== matlab function ModelRiki/Ctrl/AltCalculator/MATLAB Function ==
  data: pressure input; alt output; pressure0 input
function alt = fcn(pressure, pressure0)
%#codegen
if (pressure < 10000) || (pressure > 150000) % pressure not valid?
    alt = single(0);
else
    alt = 44330*(1-(pressure/pressure0)^(1/5.255));    
end
